simulink subsystem "Throttle_Map_2WD_NO_REGEN"  (R2023b)
settings: Solver=VariableStepAuto  StartTime=0.0  StopTime=10.0  RelTol=1e-3
undefined symbols (not defined in the file): tvs
settings Model: Creator=Inver  LastModifiedBy=Inver

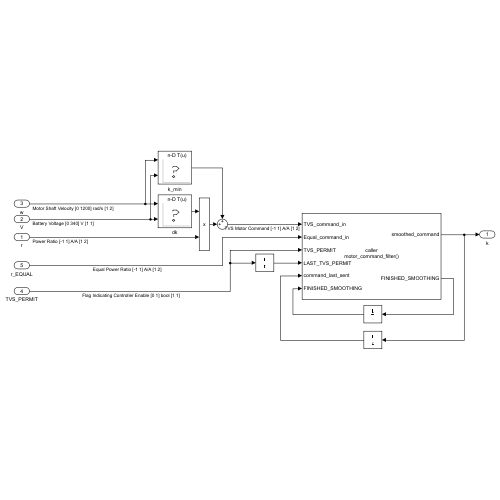
[thumbnail: Simulink's stored preview of the top-level diagram]
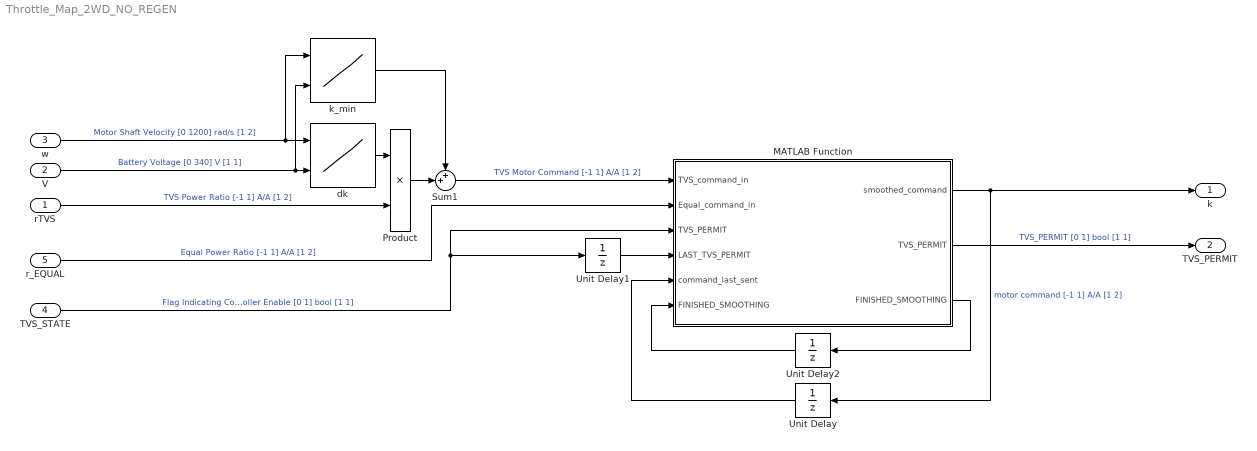
== system Throttle_Map_2WD_NO_REGEN ==
  rTVS : Inport
  V : Inport  Port=2
  w : Inport  Port=3
  TVS_STATE : Inport  Port=4
  r_EQUAL : Inport  Port=5
  MATLAB Function : MATLAB Function  TreatAsAtomicUnit=on
  Product : Product
  Sum1 : Sum  Inputs=++|
  Unit Delay : UnitDelay  InitialCondition=tvs.ic.k  SampleTime=-1  HasFrameUpgradeWarning=on
  Unit Delay1 : UnitDelay  InitialCondition=tvs.ic.LAST_TVS_PERMIT  SampleTime=-1  HasFrameUpgradeWarning=on
  Unit Delay2 : UnitDelay  InitialCondition=tvs.ic.FINISHED_SMOOTHENING  SampleTime=-1  HasFrameUpgradeWarning=on
  dk : Lookup_n-D  LookupTableObject=''  BreakpointsForDimension1=tvs.bp.w  BreakpointsForDimension2=tvs.bp.V  BreakpointsForDimension1FirstPoint=10  BreakpointsForDimension2FirstPoint=10  BreakpointsForDimension1Spacing=12  BreakpointsForDimension2Spacing=12  IndexSearchMethod=Evenly spaced points  Table=tvs.tbl.dk  ExtrapMethod=Clip  DiagnosticForOutOfRangeInput=Error  RemoveProtectionInput=on  UseLastTableValue=on  InternalRulePriority=Speed  RndMeth=Simplest
      settings: InputPortMap=u0,u1
  k_min : Lookup_n-D  LookupTableObject=''  BreakpointsForDimension1=tvs.bp.w  BreakpointsForDimension2=tvs.bp.V  BreakpointsForDimension1FirstPoint=10  BreakpointsForDimension2FirstPoint=10  BreakpointsForDimension1Spacing=12  BreakpointsForDimension2Spacing=12  IndexSearchMethod=Evenly spaced points  Table=tvs.tbl.k_min  ExtrapMethod=Clip  DiagnosticForOutOfRangeInput=Error  RemoveProtectionInput=on  UseLastTableValue=on  InternalRulePriority=Speed  RndMeth=Simplest
      settings: InputPortMap=u0,u1
  k : Outport
  TVS_PERMIT : Outport  Port=2
  wires:
  w/1 -> dk/1, k_min/1  "Motor Shaft Velocity [0 1200] rad/s [1 2]"
  V/1 -> dk/2, k_min/2  "Battery Voltage [0 340] V [1 1]"
  rTVS/1 -> Product/2  "TVS Power Ratio [-1 1] A/A [1 2]"
  Sum1/1 -> MATLAB Function/1(TVS_command_in)  "TVS Motor Command [-1 1] A/A [1 2]"
  k_min/1 -> Sum1/1
  dk/1 -> Product/1
  Product/1 -> Sum1/2
  TVS_STATE/1 -> MATLAB Function/3("TVS_PERMIT "), Unit Delay1/1  "Flag Indicating Controller Enable [0 1] bool [1 1]"
  r_EQUAL/1 -> MATLAB Function/2(Equal_command_in)  "Equal Power Ratio [-1 1] A/A [1 2]"
  MATLAB Function/1(smoothed_command) -> k/1, Unit Delay/1  "motor command [-1 1] A/A [1 2]"
  Unit Delay/1 -> MATLAB Function/5(command_last_sent)
  MATLAB Function/3(FINISHED_SMOOTHING) -> Unit Delay2/1
  Unit Delay2/1 -> MATLAB Function/6("FINISHED_SMOOTHING ")
  Unit Delay1/1 -> MATLAB Function/4(LAST_TVS_PERMIT)
  MATLAB Function/2(TVS_PERMIT) -> TVS_PERMIT/1  "TVS_PERMIT [0 1] bool [1 1]"

== matlab function Throttle_Map_2WD_NO_REGEN/MATLAB Function ==
  data: TVS_command_in input size=[ 1 2]; smoothed_command output size=[1 2]; TVS_PERMIT output; Equal_command_in input size=[1 2]; TVS_PERMIT input; LAST_TVS_PERMIT input; command_last_sent input size=[1 2]; FINISHED_SMOOTHING input; FINISHED_SMOOTHING output
function [smoothed_command,TVS_PERMIT,FINISHED_SMOOTHING] = wrapper(TVS_command_in,Equal_command_in,TVS_PERMIT,LAST_TVS_PERMIT,command_last_sent,FINISHED_SMOOTHING)

    [smoothed_command,TVS_PERMIT,FINISHED_SMOOTHING] = motor_command_filter(TVS_command_in, ...
        Equal_command_in,TVS_PERMIT,LAST_TVS_PERMIT,command_last_sent,FINISHED_SMOOTHING);

end
